simulink model "lab4"  (R2017a)
settings: Solver=VariableStepAuto  StartTime=0.0  StopTime=200  RelTol=1e-3
settings Model: Creator=Priyesh  LastModifiedBy=Priyesh

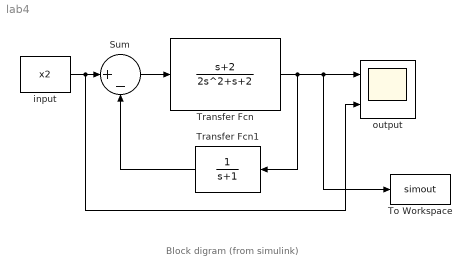
== system lab4 ==
  note: Block digram (from simulink)
  Sum : Sum  Inputs=|+-
  To Workspace : ToWorkspace  VariableName=simout  SampleTime=-1
  Transfer Fcn : TransferFcn  Numerator=[1 2]  Denominator=[2 1 2]
  Transfer Fcn1 : TransferFcn  Denominator=[1 1]
  input : FromWorkspace  VariableName=x2  SampleTime=0.001
  output : Scope  NumInputPorts=2
  wires:
  Sum/1 -> Transfer Fcn/1
  Transfer Fcn1/1 -> Sum/2
  Transfer Fcn/1 -> output/1, To Workspace/1, Transfer Fcn1/1
  input/1 -> output/2, Sum/1
